simulink model "simulink_group21"  (R2023b)
settings: Solver=FixedStepAuto  StartTime=0.0  StopTime=40.0  FixedStep=1e-3  RelTol=1e-3  EnableMultiTasking=on
undefined symbols (not defined in the file): D0, D1, D10, D11, D12, D13, D2, D3, D4, D5, D6, D7, D8, D9, PTA0, PTA1, PTA2, PTB23, PTB9, PTC16, PTC17, PTC2, PTC3, PTC4, PTD0, PTD1, PTD2, PTD3
libraries: frdmk64flib x16
settings Model: ExtModeTrigDuration=5  Creator=sadeg  LastModifiedBy=sadeg
settings OptimizationCC: EnhancedBackFolding=on  PassReuseOutputArgsThreshold=0  MaxStackSize=64  OptimizeBlockOrder=speed  DifferentSizesBufferReuse=on  OptimizationCustomize=off
settings DebuggingCC: ParameterTunabilityLossMsg=error
settings HardwareCC: ProdBitPerPointer=32  ProdBitPerSizeT=32  ProdBitPerPtrDiffT=32  ProdLargestAtomicInteger=Long  ProdLargestAtomicFloat=Double  ProdWordSize=32  ProdHWDeviceType=ARM Compatible->ARM Cortex  UseEmbeddedCoderFeatures=off
settings SFSimCC: MATLABDynamicMemAlloc=off
settings RTWCC: Description=Embedded Coder  SystemTargetFile=ert.tlc  HardwareBoard=NXP FRDM-K64F  TLCOptions="-aInlineSetEventsForThisBaseRateFcn=TLC_FALSE -aSuppressMultiTaskScheduler=TLC_FALSE  -aRateBasedStepFcn=0"  TemplateMakefile=ert_default_tmf  Toolchain=GNU Tools for ARM Embedded Processors
settings CodeAppCC: ForceParamTrailComments=on  OperatorAnnotations=on
settings ERTTargetCC: ERTCustomFileBanners=off  SupportContinuousTime=on  SupportNonInlinedSFcns=on  RemoveResetFunc=off  ModelStepFunctionPrototypeControlCompliant=off  ExtModeTransport=4  ExtModeMexFile=sendToCommService

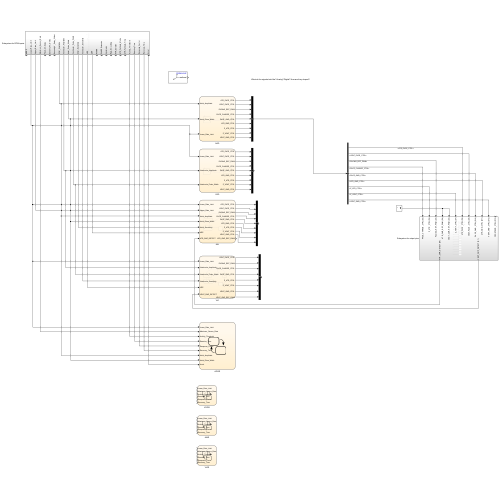
[thumbnail: Simulink's stored preview of the top-level diagram]
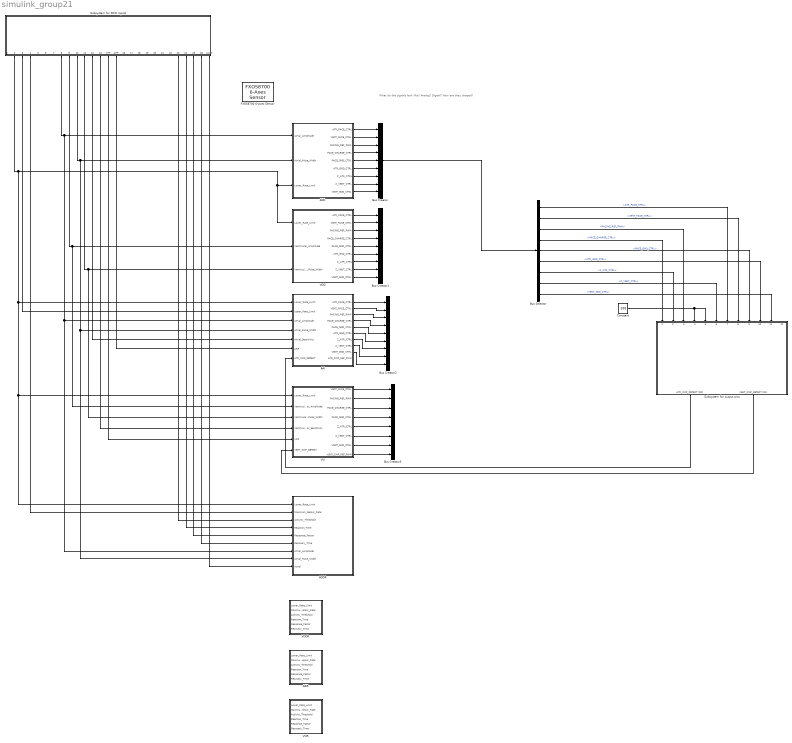
== system simulink_group21 ==
  note: What do the signals look like? Analog? Digital? How are they shaped?
  AAI : Stateflow chart  TreatAsAtomicUnit=on
  AAIR : Stateflow chart  TreatAsAtomicUnit=on
      settings: PortSchema="{\"entries\":[{\"content\":{\"sides\":[{\"content\":{\"connectorIds\":[\"In1\",\"In2\",\"In3\",\"In6\",\"In4\",\"In5\"]},\"type\":\"ConnectorPlacement.EquallySpacedRectSide\",\"uuid\":\"e09ad94b-7f01-4c3c-a94c-93cb9f7cca8b\"},{\"content\":{\"side\":\"RIGHT\"},\"type\":\"ConnectorPlacement.EquallySpacedRectSide\",\"uuid\":\"328884ea-f542-4d2b-921c-41d38e86bf3b\"},{\"content\":{\"side\":\"TOP\"},\"type\":\"ConnectorPlacement.EquallySpacedRectSide\",\"uuid\":\"67f800ab-4ed8-4490-8840-21364fa6510e\"}]},\"type\":\"ConnectorPlacement.EquallySpacedConnector\",\"uuid\":\"0d54d946-90a5-43e4-96eb-61bef4d09b17\"}],\"packageUris\":[\"http://schema.mathworks.com/mf0/Connector/R2020b\"],\"version\":\"1.0\"}"
  AOO : Stateflow chart  TreatAsAtomicUnit=on
      settings: PortSchema="{\"entries\":[{\"content\":{\"sides\":[{\"content\":{\"connectorIds\":[\"In1\",\"In2\",\"In3\"]},\"type\":\"ConnectorPlacement.EquallySpacedRectSide\",\"uuid\":\"492a7fcf-0136-4cc6-a368-2e6eb8f4a8f6\"},{\"content\":{\"connectorIds\":[\"Out1\",\"Out2\",\"Out3\",\"Out4\",\"Out5\",\"Out8\",\"Out6\",\"Out7\",\"Out9\"],\"side\":\"RIGHT\"},\"type\":\"ConnectorPlacement.EquallySpacedRectSide\",\"uuid\":\"446f1639-51dc-43c3-8eec-8a39ae78ded7\"},{\"content\":{\"side\":\"TOP\"},\"type\":\"ConnectorPlacement.EquallySpacedRectSide\",\"uuid\":\"77fd6d12-343c-45d8-9399-9fe0379be2cf\"}]},\"type\":\"ConnectorPlacement.EquallySpacedConnector\",\"uuid\":\"42a5ffd8-4660-4821-97a9-3a811e8cbc3e\"}],\"packageUris\":[\"http://schema.mathworks.com/mf0/Connector/R2020b\"],\"version\":\"1.0\"}"
  AOOR : Stateflow chart  TreatAsAtomicUnit=on
      settings: PortSchema="{\"entries\":[{\"content\":{\"sides\":[{\"content\":{\"connectorIds\":[\"In1\",\"In2\",\"In3\",\"In6\",\"In4\",\"In5\",\"In8\",\"In7\",\"In9\"]},\"type\":\"ConnectorPlacement.EquallySpacedRectSide\",\"uuid\":\"e09ad94b-7f01-4c3c-a94c-93cb9f7cca8b\"},{\"content\":{\"side\":\"RIGHT\"},\"type\":\"ConnectorPlacement.EquallySpacedRectSide\",\"uuid\":\"328884ea-f542-4d2b-921c-41d38e86bf3b\"},{\"content\":{\"side\":\"TOP\"},\"type\":\"ConnectorPlacement.EquallySpacedRectSide\",\"uuid\":\"67f800ab-4ed8-4490-8840-21364fa6510e\"}]},\"type\":\"ConnectorPlacement.EquallySpacedConnector\",\"uuid\":\"0d54d946-90a5-43e4-96eb-61bef4d09b17\"}],\"packageUris\":[\"http://schema.mathworks.com/mf0/Connector/R2020b\"],\"version\":\"1.0\"}"
  Bus Creator : BusCreator  Inputs=9
  Bus Creator1 : BusCreator  Inputs=9
  Bus Creator2 : BusCreator  Inputs=9
  Bus Creator3 : BusCreator  Inputs=8
  Bus Selector : BusSelector  OutputSignals=ATR_PACE_CTRL,VENT_PACE_CTRL,PACING_REF_PWM,PACE_CHARGE_CTRL,PACE_GND_CTRL,ATR_GND_CTRL,Z_ATR_CTRL,Z_VENT_CTRL,VENT_GND_CTRL
  Constant : Constant  Value=100
  FXOS8700 6-Axes Sensor : frdmk64flib/FXOS8700 6-Axes Sensor  Activesensor=Accelerometer only  ODR=800Hz  HybridODR=400Hz  Accelfullrange=-4g to +4g  SampleTime=-1
  Subsystem for DCM inputs : Subsystem
  Subsystem for output pins : Subsystem
  VOO : Stateflow chart  TreatAsAtomicUnit=on
  VOOR : Stateflow chart  TreatAsAtomicUnit=on
      settings: PortSchema="{\"entries\":[{\"content\":{\"sides\":[{\"content\":{\"connectorIds\":[\"In1\",\"In2\",\"In3\",\"In6\",\"In4\",\"In5\"]},\"type\":\"ConnectorPlacement.EquallySpacedRectSide\",\"uuid\":\"e09ad94b-7f01-4c3c-a94c-93cb9f7cca8b\"},{\"content\":{\"side\":\"RIGHT\"},\"type\":\"ConnectorPlacement.EquallySpacedRectSide\",\"uuid\":\"328884ea-f542-4d2b-921c-41d38e86bf3b\"},{\"content\":{\"side\":\"TOP\"},\"type\":\"ConnectorPlacement.EquallySpacedRectSide\",\"uuid\":\"67f800ab-4ed8-4490-8840-21364fa6510e\"}]},\"type\":\"ConnectorPlacement.EquallySpacedConnector\",\"uuid\":\"0d54d946-90a5-43e4-96eb-61bef4d09b17\"}],\"packageUris\":[\"http://schema.mathworks.com/mf0/Connector/R2020b\"],\"version\":\"1.0\"}"
  VVI : Stateflow chart  TreatAsAtomicUnit=on
  VVIR : Stateflow chart  TreatAsAtomicUnit=on
      settings: PortSchema="{\"entries\":[{\"content\":{\"sides\":[{\"content\":{\"connectorIds\":[\"In1\",\"In2\",\"In3\",\"In6\",\"In4\",\"In5\"]},\"type\":\"ConnectorPlacement.EquallySpacedRectSide\",\"uuid\":\"e09ad94b-7f01-4c3c-a94c-93cb9f7cca8b\"},{\"content\":{\"side\":\"RIGHT\"},\"type\":\"ConnectorPlacement.EquallySpacedRectSide\",\"uuid\":\"328884ea-f542-4d2b-921c-41d38e86bf3b\"},{\"content\":{\"side\":\"TOP\"},\"type\":\"ConnectorPlacement.EquallySpacedRectSide\",\"uuid\":\"67f800ab-4ed8-4490-8840-21364fa6510e\"}]},\"type\":\"ConnectorPlacement.EquallySpacedConnector\",\"uuid\":\"0d54d946-90a5-43e4-96eb-61bef4d09b17\"}],\"packageUris\":[\"http://schema.mathworks.com/mf0/Connector/R2020b\"],\"version\":\"1.0\"}"
  wires:
  Subsystem for DCM inputs/2(Lower_Rate_Limit) -> AOO/3(Lower_Rate_Limit), VOO/1(Lower_Rate_Limit), AAI/1(Lower_Rate_Limit), AOOR/1(Lower_Rate_Limit), VVI/1(Lower_Rate_Limit)
  Subsystem for DCM inputs/3(Upper_Rate_Limit) -> AAI/2(Upper_Rate_Limit)
  Subsystem for DCM inputs/8(Atrial_Amplitude) -> AAI/3(Atrial_Amplitude), AOOR/8(Atrial_Amplitude), AOO/1(Atrial_Amplitude)
  Subsystem for DCM inputs/10(Atrial_Pulse_Width) -> AAI/4(Atrial_Pulse_Width), AOOR/7(Atrial_Pulse_Width), AOO/2(Atrial_Pulse_Width)
  Subsystem for DCM inputs/9(Ventricular_Amplitude) -> VOO/2(Ventricular_Amplitude), VVI/2(Ventricular_Amplitude)
  Subsystem for DCM inputs/11(Ventricular_Pulse_Width) -> VOO/3(Ventricular_Pulse_Width), VVI/3(Ventricular_Pulse_Width)
  Subsystem for DCM inputs/12(Atrial_Sensitivity) -> AAI/5(Atrial_Sensitivity)
  Subsystem for DCM inputs/15(ARP) -> AAI/6(ARP)
  Subsystem for DCM inputs/13(Ventricular_Sensitivity) -> VVI/4(Ventricular_Sensitivity)
  Subsystem for DCM inputs/14(VRP) -> VVI/5(VRP)
  AOO/1(ATR_PACE_CTRL) -> Bus Creator/1
  AOO/2(VENT_PACE_CTRL) -> Bus Creator/2
  AOO/3(PACING_REF_PWM) -> Bus Creator/3
  AOO/4(PACE_CHARGE_CTRL) -> Bus Creator/4
  AOO/5(PACE_GND_CTRL) -> Bus Creator/5
  AOO/8(ATR_GND_CTRL) -> Bus Creator/6
  AOO/6(Z_ATR_CTRL) -> Bus Creator/7
  AOO/7(Z_VENT_CTRL) -> Bus Creator/8
  AOO/9(VENT_GND_CTRL) -> Bus Creator/9
  VOO/1(ATR_PACE_CTRL) -> Bus Creator1/1
  VOO/2(VENT_PACE_CTRL) -> Bus Creator1/2
  VOO/3(PACING_REF_PWM) -> Bus Creator1/3
  VOO/4(PACE_CHARGE_CTRL) -> Bus Creator1/4
  VOO/5(PACE_GND_CTRL) -> Bus Creator1/5
  VOO/6(ATR_GND_CTRL) -> Bus Creator1/6
  VOO/7(Z_ATR_CTRL) -> Bus Creator1/7
  VOO/8(Z_VENT_CTRL) -> Bus Creator1/8
  VOO/9(VENT_GND_CTRL) -> Bus Creator1/9
  AAI/9(VENT_GND_CTRL) -> Bus Creator2/9
  AAI/2(VENT_PACE_CTRL) -> Bus Creator2/2
  AAI/1(ATR_PACE_CTRL) -> Bus Creator2/1
  AAI/4(PACE_CHARGE_CTRL) -> Bus Creator2/4
  AAI/6(ATR_GND_CTRL) -> Bus Creator2/6
  AAI/3(PACING_REF_PWM) -> Bus Creator2/3
  AAI/7(Z_ATR_CTRL) -> Bus Creator2/7
  AAI/8(Z_VENT_CTRL) -> Bus Creator2/8
  AAI/5(PACE_GND_CTRL) -> Bus Creator2/5
  VVI/7(VENT_GND_CTRL) -> Bus Creator3/7
  VVI/1(VENT_PACE_CTRL) -> Bus Creator3/1
  VVI/3(PACE_CHARGE_CTRL) -> Bus Creator3/3
  VVI/2(PACING_REF_PWM) -> Bus Creator3/2
  VVI/5(Z_ATR_CTRL) -> Bus Creator3/5
  VVI/6(Z_VENT_CTRL) -> Bus Creator3/6
  VVI/4(PACE_GND_CTRL) -> Bus Creator3/4
  Bus Selector/1 -> Subsystem for output pins/7(ATR_PACE_CTRL (D8))  "<ATR_PACE_CTRL>"
  Bus Selector/2 -> Subsystem for output pins/8(VENT_PACE_CTRL (D9))  "<VENT_PACE_CTRL>"
  Bus Selector/3 -> Subsystem for output pins/3(PACING_REF_PWM (D5))  "<PACING_REF_PWM>"
  Bus Selector/4 -> Subsystem for output pins/1(PACE_CHARGE_CTRL (D2))  "<PACE_CHARGE_CTRL>"
  Bus Selector/5 -> Subsystem for output pins/9(PACE_GND_CTRL (D10))  "<PACE_GND_CTRL>"
  Bus Selector/6 -> Subsystem for output pins/10(ATR_GND_CTRL (D11))  "<ATR_GND_CTRL>"
  Bus Selector/7 -> Subsystem for output pins/2(Z_ATR_CTRL (D4))  "<Z_ATR_CTRL>"
  Bus Selector/8 -> Subsystem for output pins/6(Z_VENT_CTRL (D7))  "<Z_VENT_CTRL>"
  Bus Selector/9 -> Subsystem for output pins/11(VENT_GND_CTRL (D12))  "<VENT_GND_CTRL>"
  VVI/8(VENT_CMP_REF_PWM) -> Bus Creator3/8
  Subsystem for output pins/2(VENT_CMP_DETECT (D1)) -> VVI/6(VENT_CMP_DETECT)
  Subsystem for output pins/1(ATR_CMP_DETECT (D0)) -> AAI/7(ATR_CMP_DETECT)
  Constant/1 -> Subsystem for output pins/4(ATR_CMP_REF_PWM (D6)), Subsystem for output pins/5(VENT_CMP_REF_PWM (D3))
  Subsystem for DCM inputs/4(Maximum_Sensor_Rate) -> AOOR/2(Maximum_Sensor_Rate)
  Subsystem for DCM inputs/23(Activity_Threshold) -> AOOR/3(Activity_Threshold)
  Subsystem for DCM inputs/24(Reaction_Time) -> AOOR/6(Reaction_Time)
  Subsystem for DCM inputs/25(Response_Factor) -> AOOR/4(Response_Factor)
  Subsystem for DCM inputs/26(Recovery_Time) -> AOOR/5(Recovery_Time)
  Bus Creator/1 -> Bus Selector/1
  Subsystem for DCM inputs/27(Accel) -> AOOR/9(Accel)

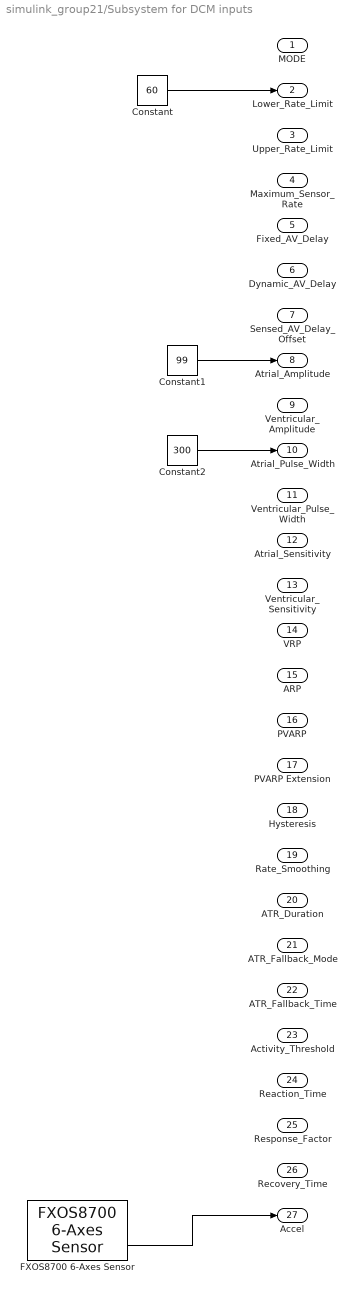
== system simulink_group21/Subsystem for DCM inputs ==
  Constant : Constant  Value=60
  Constant1 : Constant  Value=99
  Constant2 : Constant  Value=300
  FXOS8700 6-Axes Sensor : frdmk64flib/FXOS8700 6-Axes Sensor  Activesensor=Accelerometer and Magnetometer  ODR=800Hz  HybridODR=400Hz  Accelfullrange=-4g to +4g  SampleTime=-1
  MODE : Outport
  Lower_Rate_Limit : Outport  Port=2
  Upper_Rate_Limit : Outport  Port=3
  Maximum_Sensor_Rate : Outport  Port=4
  Fixed_AV_Delay : Outport  Port=5
  Dynamic_AV_Delay : Outport  Port=6
  Sensed_AV_Delay_Offset : Outport  Port=7
  Atrial_Amplitude : Outport  Port=8
  Ventricular_Amplitude : Outport  Port=9
  Atrial_Pulse_Width : Outport  Port=10
  Ventricular_Pulse_Width : Outport  Port=11
  Atrial_Sensitivity : Outport  Port=12
  Ventricular_Sensitivity : Outport  Port=13
  VRP : Outport  Port=14
  ARP : Outport  Port=15
  PVARP : Outport  Port=16
  PVARP Extension : Outport  Port=17
  Hysteresis : Outport  Port=18
  Rate_Smoothing : Outport  Port=19
  ATR_Duration : Outport  Port=20
  ATR_Fallback_Mode : Outport  Port=21
  ATR_Fallback_Time : Outport  Port=22
  Activity_Threshold : Outport  Port=23
  Reaction_Time : Outport  Port=24
  Response_Factor : Outport  Port=25
  Recovery_Time : Outport  Port=26
  Accel : Outport  Port=27
  wires:
  Constant/1 -> Lower_Rate_Limit/1
  Constant1/1 -> Atrial_Amplitude/1
  Constant2/1 -> Atrial_Pulse_Width/1
  FXOS8700 6-Axes Sensor/2 -> Accel/1

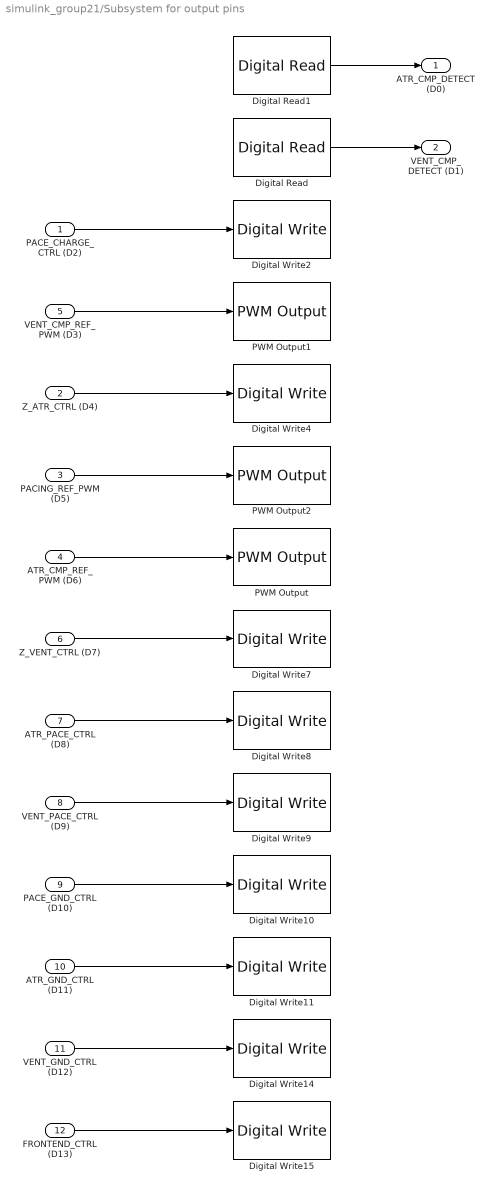
== system simulink_group21/Subsystem for output pins ==
  PACE_CHARGE_CTRL (D2) : Inport
  Z_ATR_CTRL (D4) : Inport  Port=2
  PACING_REF_PWM (D5) : Inport  Port=3
  ATR_CMP_REF_PWM (D6) : Inport  Port=4
  VENT_CMP_REF_PWM (D3) : Inport  Port=5
  Z_VENT_CTRL (D7) : Inport  Port=6
  ATR_PACE_CTRL (D8) : Inport  Port=7
  VENT_PACE_CTRL (D9) : Inport  Port=8
  PACE_GND_CTRL (D10) : Inport  Port=9
  ATR_GND_CTRL (D11) : Inport  Port=10
  VENT_GND_CTRL (D12) : Inport  Port=11
  FRONTEND_CTRL (D13) : Inport  Port=12
  Digital Read : frdmk64flib/Digital Read  Whichpin=PTC17 (D1)  SampleTime=-1
  Digital Read1 : frdmk64flib/Digital Read  Whichpin=PTC16 (D0)  SampleTime=-1
  Digital Write10 : frdmk64flib/Digital Write  Whichpin=PTD0 (D10)
  Digital Write11 : frdmk64flib/Digital Write  Whichpin=PTD2 (D11)
  Digital Write14 : frdmk64flib/Digital Write  Whichpin=PTD3 (D12)
  Digital Write15 : frdmk64flib/Digital Write  Whichpin=PTD1 (D13)
  Digital Write2 : frdmk64flib/Digital Write  Whichpin=PTB9 (D2)
  Digital Write4 : frdmk64flib/Digital Write  Whichpin=PTB23 (D4)
  Digital Write7 : frdmk64flib/Digital Write  Whichpin=PTC3 (D7)
  Digital Write8 : frdmk64flib/Digital Write  Whichpin=PTA0 (D8)
  Digital Write9 : frdmk64flib/Digital Write  Whichpin=PTC4 (D9)
  PWM Output : frdmk64flib/PWM Output  Whichpin=PTC2 (D6)  InitialFrequency=2000  InitialDutyCycle=0
  PWM Output1 : frdmk64flib/PWM Output  Whichpin=PTA1 (D3)  InitialFrequency=2000  InitialDutyCycle=0
  PWM Output2 : frdmk64flib/PWM Output  Whichpin=PTA2 (D5)  InitialFrequency=2000  InitialDutyCycle=0
  ATR_CMP_DETECT (D0) : Outport
  VENT_CMP_DETECT (D1) : Outport  Port=2
  wires:
  PACE_CHARGE_CTRL (D2)/1 -> Digital Write2/1
  Z_ATR_CTRL (D4)/1 -> Digital Write4/1
  VENT_CMP_REF_PWM (D3)/1 -> PWM Output1/1
  PACING_REF_PWM (D5)/1 -> PWM Output2/1
  Z_VENT_CTRL (D7)/1 -> Digital Write7/1
  ATR_CMP_REF_PWM (D6)/1 -> PWM Output/1
  PACE_GND_CTRL (D10)/1 -> Digital Write10/1
  ATR_GND_CTRL (D11)/1 -> Digital Write11/1
  ATR_PACE_CTRL (D8)/1 -> Digital Write8/1
  VENT_PACE_CTRL (D9)/1 -> Digital Write9/1
  VENT_GND_CTRL (D12)/1 -> Digital Write14/1
  FRONTEND_CTRL (D13)/1 -> Digital Write15/1
  Digital Read/1 -> VENT_CMP_DETECT (D1)/1
  Digital Read1/1 -> ATR_CMP_DETECT (D0)/1

== stateflow chart simulink_group21/AOO ==
  note: AOO: Pace Atrium at constant rate
  state DISCHARGE
    during:
    %Discharge C22 into Atrium
    %Begin Charging C21 Blocking Capacitor
    PACE_CHARGE_CTRL = 0;
    PACE_GND_CTRL = 1;
    ATR_PACE_CTRL = 1;
    ATR_GND_CTRL = 0;
    Z_ATR_CTRL = 0;
    Z_VENT_CTRL = 0;
    VENT_GND_CTRL = 0;
    VENT_PACE_CTRL  = 0;
  state CHARGE
    during:
    % Start Charging C22
    ATR_PACE_CTRL = 0;
    VENT_PACE_CTRL = 0;
    PACING_REF_PWM = Atrial_Amplitude
    PACE_CHARGE_CTRL = 1;
    %Begin Discharging C21 Blocking Capacitor
    PACE_GND_CTRL = 1;
    VENT_PACE_CTRL = 0;
    VENT_GND_CTRL = 0;
    Z_ATR_CTRL = 0;
    Z_VENT_CTRL = 0;
    ATR_PACE_CTRL = 0;
    ATR_GND_CTRL = 1;
  (default) -> CHARGE
  CHARGE -> DISCHARGE : after((60000/Lower_Rate_Limit)- (Atrial_Pulse_Width), msec)
  DISCHARGE -> CHARGE : after(Atrial_Pulse_Width,msec)
  data: Atrial_Amplitude input; Atrial_Pulse_Width input; ATR_PACE_CTRL output; VENT_PACE_CTRL output; PACING_REF_PWM output; PACE_CHARGE_CTRL output; PACE_GND_CTRL output; Z_ATR_CTRL output; Z_VENT_CTRL output; ATR_GND_CTRL output; VENT_GND_CTRL output; Lower_Rate_Limit input

== stateflow chart simulink_group21/VVI ==
  state hold
    entry:
  note: skip pulse if natural heart beat is detected
  state PULSE_VENT
    entry:
    % C22 begins  discharging
    PACE_CHARGE_CTRL = 0;
    % C21 begins charging
    VENT_GND_CTRL = 0;
    VENT_PACE_CTRL = 1;
  state CHARGE
    entry:
    %C22 begins charging
    VENT_PACE_CTRL = 0;
    PACE_CHARGE_CTRL = 1;
  state INIT
    entry:
    VENT_CMP_REF_PWM = Ventricular_Sensitivity;
    PACING_REF_PWM = Ventricular_Amplitude;
    VENT_GND_CTRL = 0;
    VENT_PACE_CTRL = 0;
    Z_ATR_CTRL = 0;
    Z_VENT_CTRL = 0;
    PACE_GND_CTRL = 1;
  state DISCHARGE
    entry:
    %C21 begins discharging
    VENT_PACE_CTRL = 0;
    VENT_GND_CTRL = 1;
  hold -> PULSE_VENT [order 1] : after((60000/Lower_Rate_Limit) - Ventricular_Pulse_Width-VRP, msec)
  CHARGE -> hold : after(VRP, msec)
  hold -> CHARGE [order 2] : [VENT_CMP_DETECT == 1]
  INIT -> CHARGE
  PULSE_VENT -> DISCHARGE : after(Ventricular_Pulse_Width, msec)
  (default) -> INIT
  DISCHARGE -> INIT
  data: Lower_Rate_Limit input; Ventricular_Amplitude input; Ventricular_Pulse_Width input; Ventricular_Sensitivity input; VRP input; VENT_PACE_CTRL output; PACING_REF_PWM output; PACE_CHARGE_CTRL output; PACE_GND_CTRL output; Z_ATR_CTRL output; Z_VENT_CTRL output; VENT_GND_CTRL output; VENT_CMP_REF_PWM output; VENT_CMP_DETECT input

== stateflow chart simulink_group21/AOOR ==
  data: Lower_Rate_Limit input; Maximum_Sensor_Rate input; Activity_Threshold input; Response_Factor input; Recovery_Time input; Reaction_Time input; Atrial_Pulse_Width input; Atrial_Amplitude input; Accel input

== stateflow chart simulink_group21/VOOR ==
  data: Lower_Rate_Limit input; Maximum_Sensor_Rate input; Activity_Threshold input; Response_Factor input; Recovery_Time input; Reaction_Time input

== stateflow chart simulink_group21/AAIR ==
  data: Lower_Rate_Limit input; Maximum_Sensor_Rate input; Activity_Threshold input; Response_Factor input; Recovery_Time input; Reaction_Time input

== stateflow chart simulink_group21/VVIR ==
  data: Lower_Rate_Limit input; Maximum_Sensor_Rate input; Activity_Threshold input; Response_Factor input; Recovery_Time input; Reaction_Time input

== stateflow chart simulink_group21/VOO ==
  note: VOO: Pace Ventrical at constant rate
  state DISCHARGE
    during:
    %Discharge C22 into Ventrical
    %Begin Charging C21 Blocking Capacitor
    PACE_CHARGE_CTRL = 0;
    PACE_GND_CTRL = 1;
    ATR_PACE_CTRL = 0;
    ATR_GND_CTRL = 0;
    Z_ATR_CTRL = 0;
    Z_VENT_CTRL = 0;
    VENT_GND_CTRL = 0;
    VENT_PACE_CTRL  = 1;
  state CHARGE
    during:
    % Start Charging C22
    ATR_PACE_CTRL = 0;
    VENT_PACE_CTRL = 0;
    PACING_REF_PWM = Ventricular_Amplitude*20
    PACE_CHARGE_CTRL = 1;
    %Begin Discharging C21 Blocking Capacitor
    PACE_GND_CTRL = 1;
    VENT_PACE_CTRL = 0;
    VENT_GND_CTRL = 0;
    Z_ATR_CTRL = 0;
    Z_VENT_CTRL = 0;
    ATR_PACE_CTRL = 0;
    ATR_GND_CTRL = 1;
  (default) -> CHARGE
  CHARGE -> DISCHARGE : after((60/Lower_Rate_Limit) - (Ventricular_Pulse_Width/1000), sec)
  DISCHARGE -> CHARGE : after(Ventricular_Pulse_Width,msec)
  data: Lower_Rate_Limit input; Ventricular_Amplitude input; Ventricular_Pulse_Width input; ATR_PACE_CTRL output; VENT_PACE_CTRL output; PACING_REF_PWM output; PACE_CHARGE_CTRL output; PACE_GND_CTRL output; ATR_GND_CTRL output; Z_ATR_CTRL output; Z_VENT_CTRL output; VENT_GND_CTRL output

== stateflow chart simulink_group21/AAI ==
  state hold
    entry:
  note: skip pulse if natural heart beat is detected
  state CHARGE
    entry:
    %C22 begins charging
    ATR_PACE_CTRL = 0;
    PACE_CHARGE_CTRL = 1;
  state PULSE_ATR
    entry:
    % C22 begins discharging
    PACE_CHARGE_CTRL = 0;
    % C21 begins charging
    ATR_GND_CTRL = 0;
    ATR_PACE_CTRL = 1;
  note: AAI will only pace the atrium if the natural heartbeat drops below that of the defined lower limit
  state INIT
    entry:
    ATR_CMP_REF_PWM = Atrial_Sensitivity;
    PACING_REF_PWM = Atrial_Amplitude;
    VENT_GND_CTRL = 0;
    VENT_PACE_CTRL = 0;
    Z_ATR_CTRL = 0;
    Z_VENT_CTRL = 0;
    PACE_GND_CTRL = 1;
  state DISCHARGE
    entry:
    % C21 discharging
    ATR_PACE_CTRL = 0;
    ATR_GND_CTRL = 1;
  hold -> PULSE_ATR [order 1] : after((60000/Lower_Rate_Limit) - (Atrial_Pulse_Width)-ARP, msec)
  CHARGE -> hold : after(ARP, msec)
  hold -> CHARGE [order 2] : [ATR_CMP_DETECT == 1]
  INIT -> CHARGE
  PULSE_ATR -> DISCHARGE : after(Atrial_Pulse_Width, msec)
  (default) -> INIT
  DISCHARGE -> INIT
  data: Lower_Rate_Limit input; Upper_Rate_Limit input; Atrial_Amplitude input; Atrial_Pulse_Width input; Atrial_Sensitivity input; ARP input; ATR_PACE_CTRL output; VENT_PACE_CTRL output; PACING_REF_PWM output; PACE_CHARGE_CTRL output; PACE_GND_CTRL output; ATR_GND_CTRL output; Z_ATR_CTRL output; Z_VENT_CTRL output; VENT_GND_CTRL output; ATR_CMP_DETECT input; ATR_CMP_REF_PWM output
